simulink model "mdl_pm_foc_allpu"  (R2024a)
settings: Solver=FixedStepAuto  StartTime=0.0  StopTime=1  FixedStep=0.001  RelTol=1e-3
undefined symbols (not defined in the file): param, sigbuilder_block
settings Model: Creator=jack  LastModifiedBy=steve
settings SolverCC: ZeroCrossControl=DisableAll  ZeroCrossAlgorithm=Adaptive
settings OptimizationCC: ReuseModelBlockBuffer=off
settings DebuggingCC: MaskedZcDiagnostic=none  IgnoredZcDiagnostic=none
settings RTWCC: GPUComputeCapability=3.5

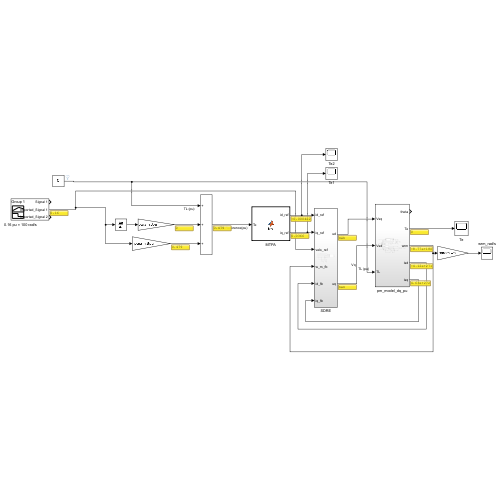
[thumbnail: Simulink's stored preview of the top-level diagram]
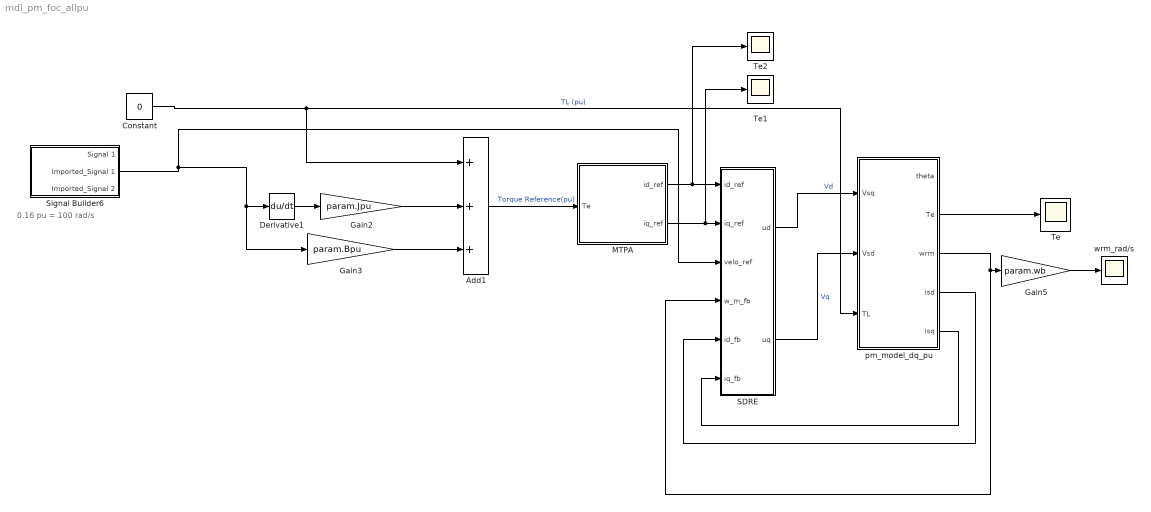
== system mdl_pm_foc_allpu ==
  note: 0.16 pu = 100 rad/s
  Add1 : Sum  Inputs=+++
  Constant : Constant  Value=0
  Derivative1 : Derivative
  Gain2 : Gain  Gain=param.Jpu
  Gain3 : Gain  Gain=param.Bpu
  Gain5 : Gain  Gain=param.wb
  MTPA : MATLAB Function  TreatAsAtomicUnit=on
  SDRE : Subsystem
  Signal Builder6 : Subsystem  Tag=STV Subsys  LoadFcn=sigbuilder_block('load');  StartFcn=sigbuilder_block('start');  StopFcn=sigbuilder_block('stop');  ClipboardFcn=sigbuilder_block('clipboard');  mask(Sigbuilder block){tuvar=[0:10]}
      mask help: Simulink:masks:SigbuilderBlock_MD
      mask init:
      | if ~strcmp(get_param(bdroot(gcbh),'SimulationStatus'),'stopped') tuvar = sigbuilder_block('maskInit'); end
      settings: CopyFcn=sigbuilder_block('copy');  DeleteFcn=sigbuilder_block('delete');  ModelCloseFcn=sigbuilder_block('modelClose');  PreSaveFcn=sigbuilder_block('preSave');  PauseFcn=sigbuilder_block('pause');  ContinueFcn=sigbuilder_block('continue');  NameChangeFcn=sigbuilder_block('namechange');  OpenFcn=sigbuilder_block('open',[481.5 164.25 551.25 399.75 ]);  CloseFcn=sigbuilder_block('close');
      mask Display: plot(0, 0, 100, 100,[2, 2, 32, 32, 2], [68, 8, 8, 68, 68],[32, 2], [38, 38], [32, 19, 2],[53, 60, 44], [32, 17, 17, 2],[16, 16, 31, 31]);txt = getActiveGroup(gcbh);text(2, 100, txt,'verticalAlignment', 'top');
  Te : Scope
  Te1 : Scope
  Te2 : Scope
  pm_model_dq_pu : Subsystem
  wrm_rad/s : Scope
  wires:
  pm_model_dq_pu/2(Te) -> Te/1
  Gain5/1 -> wrm_rad/s/1
  Constant/1 -> Add1/1, pm_model_dq_pu/3(TL)  "TL (pu)"
  Gain3/1 -> Add1/3
  Add1/1 -> MTPA/1(Te)  "Torque Reference(pu)"
  Gain2/1 -> Add1/2
  Signal Builder6/2(Imported_Signal 1) -> SDRE/3(velo_ref), Gain3/1, Derivative1/1
  MTPA/1(id_ref) -> Te2/1, SDRE/1(id_ref)
  Derivative1/1 -> Gain2/1
  MTPA/2(iq_ref) -> Te1/1, SDRE/2(iq_ref)
  SDRE/2(uq) -> pm_model_dq_pu/2(Vsd)  "Vq"
  SDRE/1(ud) -> pm_model_dq_pu/1(Vsq)  "Vd"
  pm_model_dq_pu/5(isq) -> SDRE/6(iq_fb)
  pm_model_dq_pu/3(wrm) -> SDRE/4(w_m_fb), Gain5/1
  pm_model_dq_pu/4(isd) -> SDRE/5(id_fb)

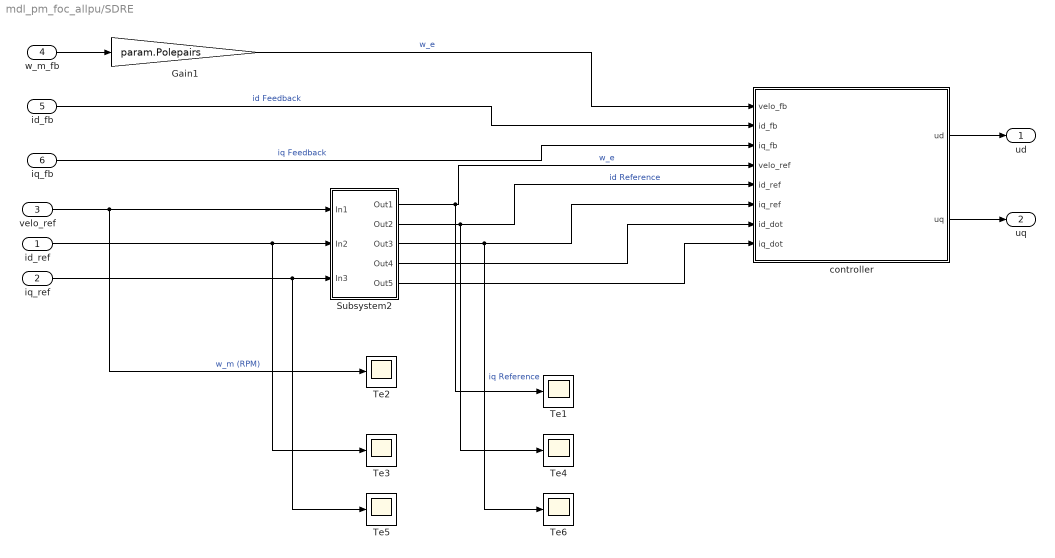
== system mdl_pm_foc_allpu/SDRE ==
  id_ref : Inport
  iq_ref : Inport  Port=2
  velo_ref : Inport  Port=3
  w_m_fb : Inport  Port=4
  id_fb : Inport  Port=5
  iq_fb : Inport  Port=6
  Gain1 : Gain  Gain=param.Polepairs
  Subsystem2 : Subsystem
  Te{1..6} (6 alike) : Scope
  controller : MATLAB Function  TreatAsAtomicUnit=on
  ud : Outport
  uq : Outport  Port=2
  wires:
  controller/2(uq) -> uq/1
  controller/1(ud) -> ud/1
  iq_ref/1 -> Te5/1, Subsystem2/3(In3)
  id_ref/1 -> Te3/1, Subsystem2/2(In2)
  velo_ref/1 -> Te2/1, Subsystem2/1(In1)  "w_m (RPM)"
  Subsystem2/5(Out5) -> controller/8(iq_dot)
  Subsystem2/4(Out4) -> controller/7(id_dot)
  Subsystem2/1(Out1) -> Te1/1, controller/4(velo_ref)  "w_e"
  Subsystem2/2(Out2) -> controller/5(id_ref), Te4/1  "id Reference"
  Subsystem2/3(Out3) -> Te6/1, controller/6(iq_ref)  "iq Reference"
  id_fb/1 -> controller/2(id_fb)  "id Feedback"
  iq_fb/1 -> controller/3(iq_fb)  "iq Feedback"
  Gain1/1 -> controller/1(velo_fb)  "w_e"
  w_m_fb/1 -> Gain1/1

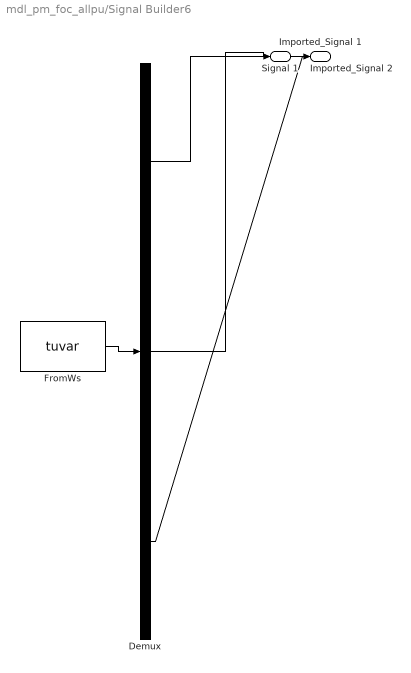
== system mdl_pm_foc_allpu/Signal Builder6 ==
  Demux : Demux  Tag=STV Demux  Outputs=3
      settings: DisplayOption=none
  FromWs : FromWorkspace  Tag=STV FromWs  VariableName=tuvar
      SigBuilderData=|
      | common.afterFinalStr = 'Extrapolate'
      | common.sampleTime = 0
      | dataSet.timeRange = [0 1]
      | dataSet.name = 'Group 1'
      | sbobj.Groups.Name = 'Group 1'
      | sbobj.Groups.Signals(1).Name = 'Signal 1'
      | sbobj.Groups.Signals(1).XData = [0 1]
      | sbobj.Groups.Signals(1).YData = [0 0]
      | sbobj.Groups.Signals(2).Name = 'Imported_Signal 1'
      | sbobj.Groups.Signals(2).XData = [0 0.1 0.4 0.46 0.52 0.58 0.8 1]
      | sbobj.Groups.Signals(2).YData = [0 0.16 0.16 0.16 0.16 0.16 0.16 0.16]
      | sbobj.Groups.Signals(3).Name = 'Imported_Signal 2'
      | sbobj.Groups.Signals(3).XData = [0 0.2 0.4 0.46 0.72 0.78 0.9 1]
      | sbobj.Groups.Signals(3).YData = [0 -900 -900 850 900 -900 -900 0]
      | sbobj.Groups.TimeRange = [0 1]
  Signal 1 : Outport  Tag=STV Outport
  Imported_Signal 1 : Outport  Tag=STV Outport  Port=2
  Imported_Signal 2 : Outport  Tag=STV Outport  Port=3
  wires:
  FromWs/1 -> Demux/1
  Demux/1 -> Signal 1/1
  Demux/2 -> Imported_Signal 1/1
  Demux/3 -> Imported_Signal 2/1

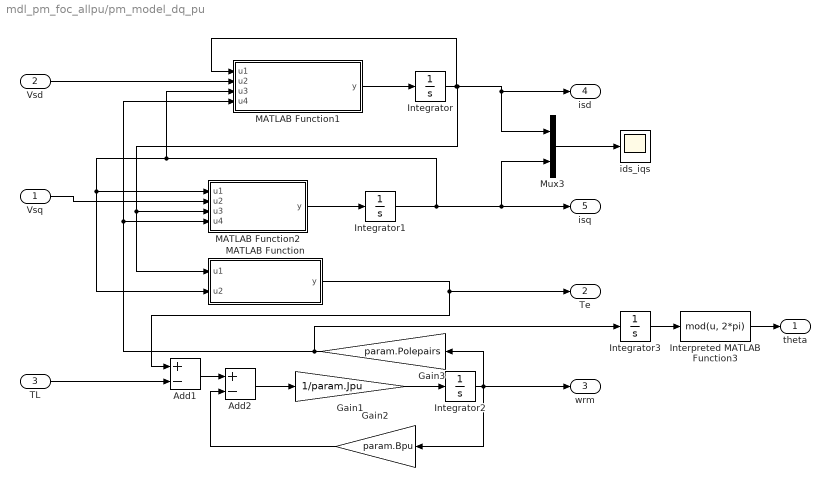
== system mdl_pm_foc_allpu/pm_model_dq_pu ==
  Vsq : Inport
  Vsd : Inport  Port=2
  TL : Inport  Port=3
  Add1 : Sum  Inputs=+-
  Add2 : Sum  Inputs=+-
  Gain1 : Gain  Gain=1/param.Jpu
  Gain2 : Gain  Gain=param.Bpu
  Gain3 : Gain  Gain=param.Polepairs
  Integrator{,1..3} (4 alike) : Integrator
  Interpreted MATLAB Function3 : MATLABFcn  MATLABFcn=mod(u, 2*pi)
  MATLAB Function : MATLAB Function  TreatAsAtomicUnit=on
  MATLAB Function1 : MATLAB Function  TreatAsAtomicUnit=on
  MATLAB Function2 : MATLAB Function  TreatAsAtomicUnit=on
  Mux3 : Mux  Inputs=2
  ids_iqs : Scope
  theta : Outport
  Te : Outport  Port=2
  wrm : Outport  Port=3
  isd : Outport  Port=4
  isq : Outport  Port=5
  wires:
  MATLAB Function2/1(y) -> Integrator1/1
  TL/1 -> Add1/2
  Vsd/1 -> MATLAB Function1/2(u2)
  Integrator1/1 -> isq/1, Mux3/2, MATLAB Function/2(u2), MATLAB Function2/1(u1), MATLAB Function1/3(u3)
  MATLAB Function/1(y) -> Te/1, Add1/1
  Gain3/1 -> Integrator3/1, MATLAB Function1/4(u4), MATLAB Function2/4(u4)
  Add2/1 -> Gain1/1
  Gain1/1 -> Integrator2/1
  Add1/1 -> Add2/1
  MATLAB Function1/1(y) -> Integrator/1
  Vsq/1 -> MATLAB Function2/2(u2)
  Integrator/1 -> MATLAB Function/1(u1), MATLAB Function2/3(u3), Mux3/1, isd/1, MATLAB Function1/1(u1)
  Integrator2/1 -> wrm/1, Gain3/1, Gain2/1
  Interpreted MATLAB Function3/1 -> theta/1
  Gain2/1 -> Add2/2
  Integrator3/1 -> Interpreted MATLAB Function3/1
  Mux3/1 -> ids_iqs/1

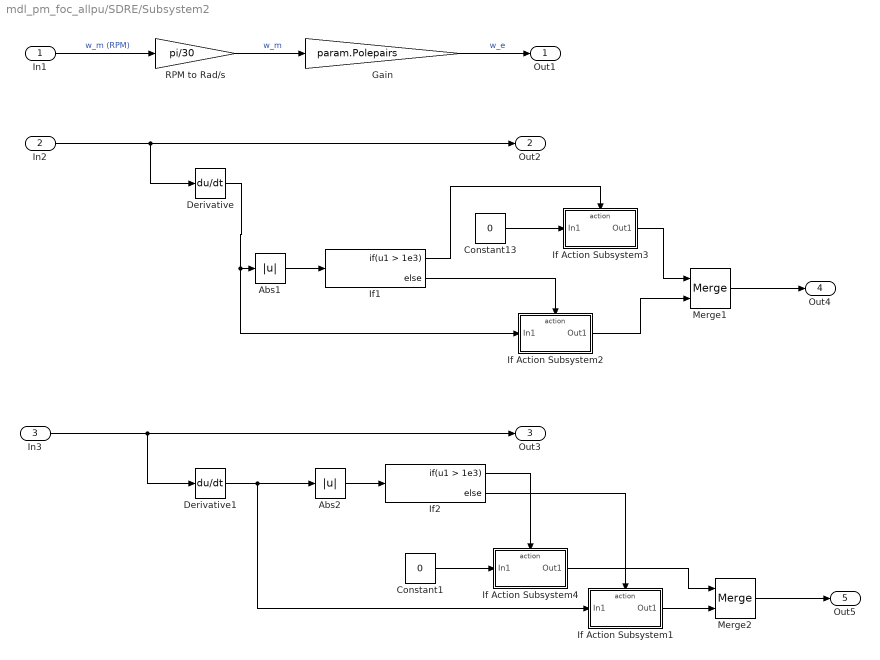
== system mdl_pm_foc_allpu/SDRE/Subsystem2 ==
  In1 : Inport
  In2 : Inport  Port=2
  In3 : Inport  Port=3
  Abs1 : Abs  SaturateOnIntegerOverflow=off
  Abs2 : Abs  SaturateOnIntegerOverflow=off
  Constant1 : Constant  Value=0
  Constant13 : Constant  Value=0
  Derivative : Derivative
  Derivative1 : Derivative
  Gain : Gain  Gain=param.Polepairs
  If Action Subsystem1 : Subsystem  TreatAsAtomicUnit=on
  If Action Subsystem2 : Subsystem  TreatAsAtomicUnit=on
  If Action Subsystem3 : Subsystem  TreatAsAtomicUnit=on
  If Action Subsystem4 : Subsystem  TreatAsAtomicUnit=on
  If1 : If  IfExpression=u1 > 1e3
  If2 : If  IfExpression=u1 > 1e3
  Merge1 : Merge
  Merge2 : Merge
  RPM to Rad/s : Gain  Gain=pi/30
  Out1 : Outport
  Out2 : Outport  Port=2
  Out3 : Outport  Port=3
  Out4 : Outport  Port=4
  Out5 : Outport  Port=5
  wires:
  Derivative1/1 -> If Action Subsystem1/1(In1), Abs2/1
  In3/1 -> Out3/1, Derivative1/1
  In1/1 -> RPM to Rad/s/1  "w_m (RPM)"
  In2/1 -> Out2/1, Derivative/1
  If Action Subsystem2/1(Out1) -> Merge1/2
  If1/1 -> If Action Subsystem3/Action
  Abs1/1 -> If1/1
  Constant13/1 -> If Action Subsystem3/1(In1)
  Derivative/1 -> If Action Subsystem2/1(In1), Abs1/1
  If1/2 -> If Action Subsystem2/Action
  If Action Subsystem3/1(Out1) -> Merge1/1
  Merge1/1 -> Out4/1
  Constant1/1 -> If Action Subsystem4/1(In1)
  If2/2 -> If Action Subsystem1/Action
  Merge2/1 -> Out5/1
  If2/1 -> If Action Subsystem4/Action
  If Action Subsystem4/1(Out1) -> Merge2/1
  If Action Subsystem1/1(Out1) -> Merge2/2
  Abs2/1 -> If2/1
  RPM to Rad/s/1 -> Gain/1  "w_m"
  Gain/1 -> Out1/1  "w_e"

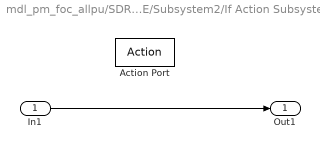
== system mdl_pm_foc_allpu/SDRE/Subsystem2/If Action Subsystem1 ==
  In1 : Inport
  Action Port : ActionPort  ActionPortLabel=else
  Out1 : Outport
  wires:
  In1/1 -> Out1/1

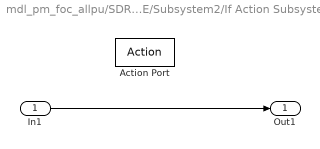
== system mdl_pm_foc_allpu/SDRE/Subsystem2/If Action Subsystem2 ==
  In1 : Inport
  Action Port : ActionPort  ActionPortLabel=else
  Out1 : Outport
  wires:
  In1/1 -> Out1/1

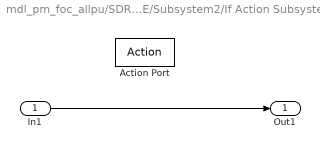
== system mdl_pm_foc_allpu/SDRE/Subsystem2/If Action Subsystem3 ==
  In1 : Inport
  Action Port : ActionPort  ActionPortLabel=if(u1 > 1e3)
  Out1 : Outport
  wires:
  In1/1 -> Out1/1

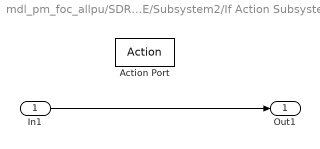
== system mdl_pm_foc_allpu/SDRE/Subsystem2/If Action Subsystem4 ==
  In1 : Inport
  Action Port : ActionPort  ActionPortLabel=if(u1 > 1e3)
  Out1 : Outport
  wires:
  In1/1 -> Out1/1

== matlab function mdl_pm_foc_allpu/pm_model_dq_pu/MATLAB Function1 ==
  data: u1 input; y output; u2 input; u3 input; u4 input; param parameter
function y = yourFunction(u1, u2, u3, u4, param)
% 從 param 結構中取出需要的參數
wb = param.wb;
Rspu = param.Rspu;
Xdpu = param.Xdpu;
Xqpu = param.Xqpu;

% 計算公式
y = -(Rspu/Xdpu)*wb*u1 + (Xqpu/Xdpu)*wb*u3*u4 + u2*wb/Xdpu;

% 容錯
if ~isfinite(y)
    y = 0;
end
end

== matlab function mdl_pm_foc_allpu/pm_model_dq_pu/MATLAB Function ==
  data: u1 input; y output; u2 input; param parameter
function y = yourFunction(u1, u2, param)
% 從 param 結構中取出需要的參數
Xdpu = param.Xdpu;
Xqpu = param.Xqpu;
Lamda_fpu = param.Lamda_fpu;


y = (Lamda_fpu * u2) + (Xdpu - Xqpu) * u1 * u2;

if ~isfinite(y)
    y = 0; % 容錯處理
end
end

== matlab function mdl_pm_foc_allpu/pm_model_dq_pu/MATLAB Function2 ==
  data: u1 input; y output; u2 input; u3 input; u4 input; param parameter
function y = yourFunction(u1, u2, u3, u4, param)

% 從 param 結構中取出需要的參數
wb = param.wb;
Rspu = param.Rspu;
Xdpu = param.Xdpu;
Xqpu = param.Xqpu;
Lamda_fpu = param.Lamda_fpu;


y = -(Rspu/Xqpu)*wb*u1 -(Xdpu/Xqpu)*wb*u3*u4 - (Lamda_fpu/Xqpu)*wb*u4 + u2*wb/Xqpu;

if ~isfinite(y)
    y = 0; % 容錯處理
end
end

== matlab function mdl_pm_foc_allpu/SDRE/controller ==
  settings: updateMethod=DISCRETE
  data: velo_fb input; id_fb input; iq_fb input; velo_ref input; id_ref input; iq_ref input; ud output; uq output; id_dot input; iq_dot input; param parameter
function [ud, uq] = SDRE_motor(velo_fb, id_fb, iq_fb, velo_ref, id_ref, iq_ref, id_dot, iq_dot, param)

% 獲取電機參數
timestep    = param.timestep;
Ld          = param.Ld;
Lq          = param.Lq;
Rs          = param.Rs;
Lamda_m     = param.Lamda_f;
pole        = param.pole;
Ib          = param.Ib;
Vb          = param.Vb;
wb          = param.wb;
Rspu        = param.Rspu;
Xdpu        = param.Xdpu;
Xqpu        = param.Xqpu;
Lamda_fpu   = param.Lamda_fpu;
Jpu         = param.Jpu;
Bpu         = param.Bpu;


persistent z_state
persistent Ts
%-------------------------------------------------------------------------------

% 初始化 z 狀態為 1
if isempty(z_state)
    z_state = 1;
end

% 自動取得取樣週期（僅限模擬模式有效）
if isempty(Ts)
    Ts = timestep;
end

% 更新 z 狀態
eta = 10;  % 衰減係數，可根據設計調整
z_state = z_state + Ts * (-eta * z_state);

%-------------------------------------------------------------------------------


if isempty(id_dot)
    id_dot = 0;
    iq_dot = 0;
end

velo_error = velo_fb - velo_ref;
id_error = id_fb - id_ref;
iq_error = iq_fb - iq_ref;

if isempty(iq_error)
    velo_error = 0;
    id_error = 0;
    iq_error = 0;
end

%-------------------------------------------------------------------------------
% 組成誤差向量（含 z 狀態）
error = [velo_error iq_error id_error z_state];

k1 = (pole*Lamda_fpu)/(2*Jpu);
k2 = Bpu/Jpu;
k3 = pole/(2*Jpu);
k4 = (wb*Rspu)/Xqpu;
k5 = (wb*Lamda_fpu)/Xqpu;
k6 = wb/Xqpu;
k7 = (wb*Rspu)/Xdpu;
k8 = wb/Xdpu;
k9 = (wb*Xqpu)/Xdpu;
k10 = (wb*Xdpu)/Xqpu;
k11 = (2*(Xdpu-Xqpu))/(2*Jpu);
% 狀態矩陣 A
A11 = -k2; 
A12 = k1; 
A13 = k11*iq_fb;

A21 = -k5-k10*id_fb; 
A22 = -k4; 
A23 = 0;

A31 = k9*iq_fb; 
A32 = 0; 
A33 = -k7;

A14 =  (1/z_state)*k11*iq_error*id_ref;
A24 = -(1/z_state)*k10*id_error*velo_ref;
A34 =  (1/z_state)*k9*iq_error*velo_ref;
A44 = - eta;

A41 = 0;
A42 = 0;
A43 = 0;

A = [A11 A12 A13 A14;
     A21 A22 A23 A24;
     A31 A32 A33 A34;
     A41 A42 A43 A44];

% 控制矩陣 B
B = [0    0;
     k6   0;
     0   k8;
     0    0];


% Q, R 矩陣
rate = sqrt(iq_error^2 + id_error^2);
Q = diag([5000, 1 + exp(-rate), 10000 + exp(-rate), 100]);  % z 的權重 100，可調
R = diag([1 1]);

%-------------------------------------------------------------------------------

% 解 SDRE 控制律
[P_ss_care, ~] = SDA_CARE(A, B, Q, R);
u_redeem = -inv(R) * B' * P_ss_care * error';

% 計算基礎電壓
ucq = (Ib*Rs/Vb) * iq_ref + (wb*Lamda_m)* velo_ref + (Ib*Lq) * iq_dot + (Ld*Ib*wb) * id_error * velo_ref + (Ld*Ib*wb) * velo_fb * id_ref;
ucd = (Ib*Rs) * id_ref + (Ib*Ld) * id_dot - (Ib*wb*Lq) * iq_error * velo_ref - (Lq*Ib*wb) * velo_fb * iq_ref;

if ucq > 1e5
    ucq = 0;
end
if ucd > 1e5
    ucd = 0;
end

% 最終控制電壓
uq = ucq + u_redeem(1);
ud = ucd + u_redeem(2);

% 保證輸出型態
ud = reshape(ud, 1, 1);
uq = reshape(uq, 1, 1);

end

== matlab function mdl_pm_foc_allpu/MTPA ==
  data: id_ref output; Te input; iq_ref output; param parameter
function [id_ref , iq_ref] = fcn(Te, param)

% 獲取電機參數
Ld          = param.Ld;
Lq          = param.Lq;
Lamda_m     = param.Lamda_f;
pole        = param.pole;
Ib          = param.Ib;
Tb          = param.Tb;

Ldq = Ld-Lq;

%Lambda_m = Lambda_m *pi/30;
p1 = 3*pole*Ldq^2 /(4*Lamda_m);
p2 = 0;
p3 = (3*pole*Lamda_m)/(4*Ib);
p4 = -(Tb/(Ib)^3)*Te;
p = [p1 p2 p3 p4];
r = roots(p);

real_solutions = r(imag(r) == 0);


iq_ref = real(max(real_solutions));
id_ref = Ib*Ldq*(iq_ref^2) /Lamda_m;
end
